simulink model "FOC_basic1_OrientedCtrl"  (R2020b)
settings: Solver=FixedStepAuto  StartTime=0.0  StopTime=inf  FixedStep=Ts  MaxStep=0.0005  RelTol=1e-3
InitFcn:
  | FOC_basic;
undefined symbols (not defined in the file): motor, Ts
libraries: mcbcontrolslib x2, autolibpmsminterior x1
settings Model: Creator=k  LastModifiedBy=k

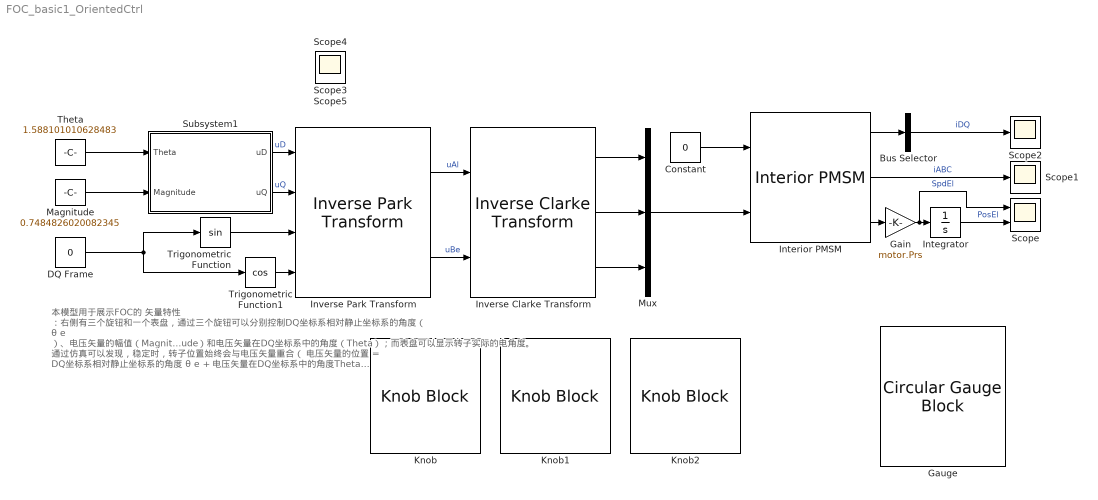
== system FOC_basic1_OrientedCtrl ==
  note: 本模型用于展示FOC的 矢量特性 ：右侧有三个旋钮和一个表盘，通过三个旋钮可以分别控制DQ坐标系相对静止坐标系的角度（ θ e ）、电压矢量的幅值（Magnitude）和电压矢量在DQ坐标系中的角度（Theta）；而表盘可以显示转子实际的电角度。
      |
      | 通过仿真可以发现，稳定时，转子位置始终会与电压矢量重合（ 电压矢量的位置 = DQ坐标系相对静止坐标系的角度 θ e + 电压矢量在DQ坐标系中的角度Theta ）。所以通合适的控制算法控制电压矢量即可控制转子的位置，这便是FOC（Field Oriented Control）的本质。
  Bus Selector : BusSelector  OutputSignals=IdSync,IqSync  OutputAsBus=on
  Constant : Constant  Value=0
  DQ Frame : Constant  Value=0
  Gain : Gain  Gain=motor.Prs
  Gauge : CircularGaugeBlock  ScaleMin=-3.14  ScaleMax=3.14  TickInterval=1.57
  Integrator : Integrator  WrapState=on
  Interior PMSM : autolibpmsminterior/Interior PMSM  port_config=Torque  sim_type=Continuous  Ts=0.001  P=motor.Prs  Rs=motor.Rs  Ldq=[motor.Ld motor.Lq]  KConstText=Permanent flux linkage constant (lambda_pm):  lambda_pm=motor.Flux  Ke=159.9771  mechanical=[motor.J, motor.B, motor.Tf]  idq0=[0 0]  theta_init=0  omega_init=0  KConst=motor.Flux  lambda_pm_calc=motor.Flux  Kt=0.07  RefBlkName='autolibpmsminterior/Interior PMSM'  aMode=5
      settings: SourceProductBaseCode=PW,MT,UV,VE,VP
  Inverse Clarke Transform : mcbcontrolslib/Inverse Clarke Transform
      settings: SourceProductBaseCode=MT
  Inverse Park Transform : mcbcontrolslib/Inverse Park Transform  AxisAlignment=D-axis
  Knob : KnobBlock  ScaleMin=-3.14  ScaleMax=3.14  TickInterval=1.57
  Knob1 : KnobBlock  ScaleMin=-12  ScaleMax=12
  Knob2 : KnobBlock  ScaleMin=-3.14  ScaleMax=3.14  TickInterval=1.57
  Magnitude : Constant  Value=0.7484826020082345
  Mux : Mux  Inputs=3
  Scope : Scope  NumInputPorts=2
  Scope{1..5} (5 alike) : Scope
  Subsystem1 : Subsystem
      mask Display: disp('Theta & Magnitue \n to Vector');
  Theta : Constant  Value=1.588101010628483
  Trigonometric Function : Trigonometry
  Trigonometric Function1 : Trigonometry  Operator=cos
  wires:
  Mux/1 -> Interior PMSM/2
  Constant/1 -> Interior PMSM/1
  DQ Frame/1 -> Trigonometric Function1/1, Trigonometric Function/1
  Interior PMSM/3 -> Gain/1
  Interior PMSM/2 -> Scope1/1  "iABC"
  Interior PMSM/1 -> Bus Selector/1
  Bus Selector/1 -> Scope2/1  "iDQ"
  Inverse Park Transform/1 -> Inverse Clarke Transform/1  "uAl"
  Inverse Park Transform/2 -> Inverse Clarke Transform/2  "uBe"
  Subsystem1/1(uD) -> Inverse Park Transform/1  "uD"
  Subsystem1/2(uQ) -> Inverse Park Transform/2  "uQ"
  Gain/1 -> Scope/1, Integrator/1  "SpdEl"
  Integrator/1 -> Scope/2  "PosEl"
  Theta/1 -> Subsystem1/1(Theta)
  Magnitude/1 -> Subsystem1/2(Magnitude)
  Inverse Clarke Transform/1 -> Mux/1
  Inverse Clarke Transform/2 -> Mux/2
  Inverse Clarke Transform/3 -> Mux/3
  Trigonometric Function1/1 -> Inverse Park Transform/4
  Trigonometric Function/1 -> Inverse Park Transform/3

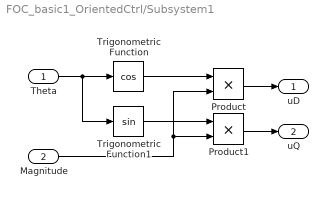
== system FOC_basic1_OrientedCtrl/Subsystem1 ==
  Theta : Inport  SampleTime=Ts
  Magnitude : Inport  Port=2  SampleTime=Ts
  Product : Product
  Product1 : Product
  Trigonometric Function : Trigonometry  Operator=cos
  Trigonometric Function1 : Trigonometry
  uD : Outport
  uQ : Outport  Port=2
  wires:
  Product/1 -> uD/1
  Product1/1 -> uQ/1
  Trigonometric Function/1 -> Product/1
  Trigonometric Function1/1 -> Product1/1
  Magnitude/1 -> Product/2, Product1/2
  Theta/1 -> Trigonometric Function1/1, Trigonometric Function/1
